simulink model "prelab"  (R2023b)
settings: Solver=VariableStepAuto  StartTime=0.0  StopTime=30  RelTol=1e-7
settings Model: Creator=Skye  LastModifiedBy=Skye

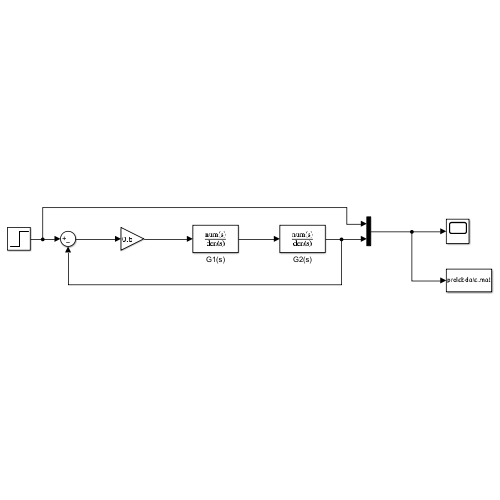
[thumbnail: Simulink's stored preview of the top-level diagram]
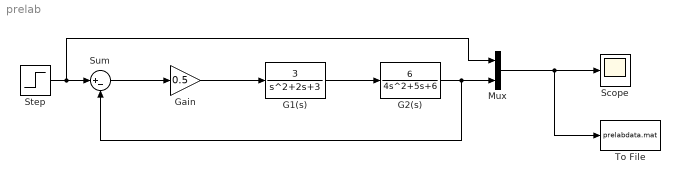
== system prelab ==
  G1(s) : TransferFcn  Numerator=[3]  Denominator=[1 2 3]
  G2(s) : TransferFcn  Numerator=[6]  Denominator=[4 5 6]
  Gain : Gain  Gain=0.5
  Mux : Mux  Inputs=2
  Scope : Scope
  Step : Step  Time=0  SampleTime=0
  Sum : Sum  Inputs=|+-
  To File : ToFile  Filename=prelabdata.mat  MatrixName=out
  wires:
  G2(s)/1 -> Sum/2, Mux/2
  G1(s)/1 -> G2(s)/1
  Gain/1 -> G1(s)/1
  Sum/1 -> Gain/1
  Step/1 -> Mux/1, Sum/1
  Mux/1 -> To File/1, Scope/1
